simulink model "basic_model_2"  (R2024b)
settings: Solver=VariableStepAuto  StartTime=0.0  StopTime=0.2  RelTol=1e-3
libraries: spsPermanentMagnetSynchronousMachineLib x1, spsDCVoltageSourceLib x1, spsGroundLib x1, spsUniversalBridgeLib x1, sps_lib x1

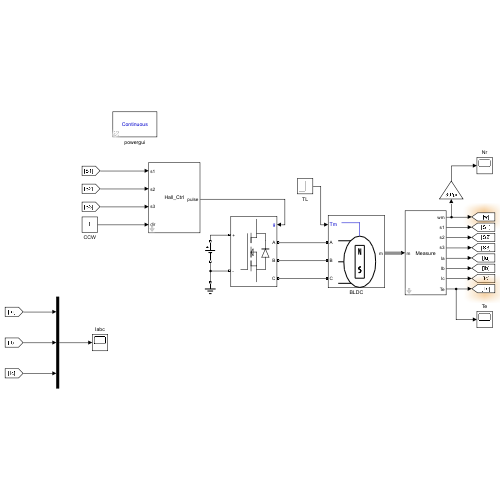
[thumbnail: Simulink's stored preview of the top-level diagram]
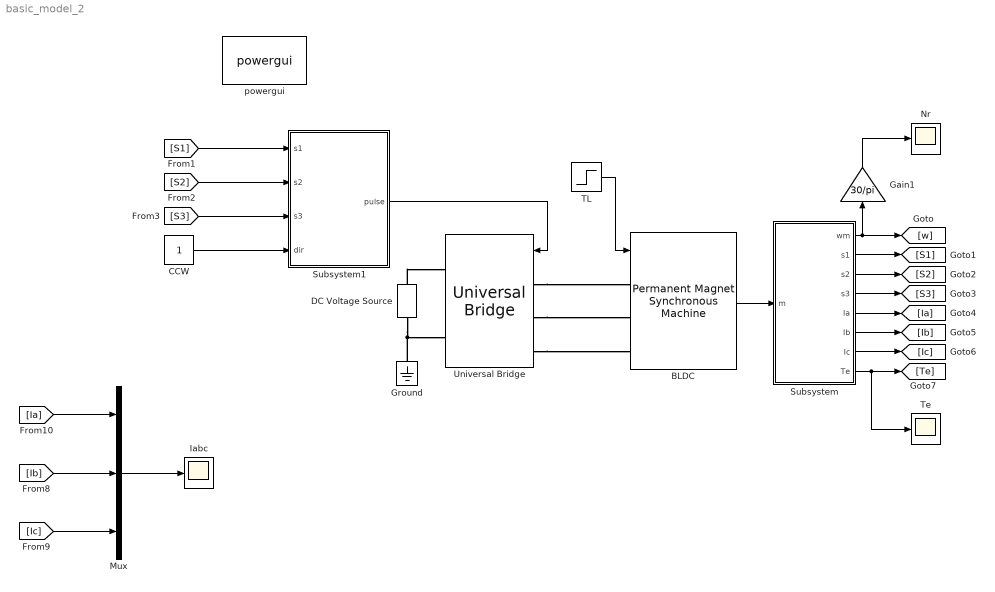
== system basic_model_2 ==
  BLDC : spsPermanentMagnetSynchronousMachineLib/Permanent Magnet Synchronous Machine  NbPhases=3  FluxDistribution=Trapezoidal  RotorType=Round  MechanicalLoad=Torque Tm  PresetModel=No  ShowDetailedParameters=on  MeasurementBus=off  Resistance=0.106/2  Inductance=0.000428/2  dqInductances=[8.5e-3,8.5e-3]  La=0.000395  MachineConstant=Torque Constant (N.m / A_peak)  Flux=0.041  VoltageCst=17.174  TorqueCst=0.164  Flat=120  Mechanical=[4943e-7 0.001 2 0]  PolePairs=4  InitialConditions=[0,0, 0,0]  InitialConditions5ph=[0 0 0 0 0 0]  RefAngle=Aligned with phase A axis (original Park)  IterativeDiscreteModel=Trapezoidal non iterative  TsBlock=-1  TsPowergui=0
  CCW : Constant
  DC Voltage Source : spsDCVoltageSourceLib/DC Voltage Source  Amplitude=50  Measurements=None
  Gain1 : Gain  Gain=30/pi
  Ground : spsGroundLib/Ground  LConnTagsString=a
  Iabc : Scope
  Mux : Mux  Inputs=3
  Nr : Scope
  Subsystem : Subsystem
  Subsystem1 : Subsystem
  TL : Step  Time=0.1  After=2  SampleTime=0
  Te : Scope
  Universal Bridge : spsUniversalBridgeLib/Universal Bridge  Arms=3  SnubberResistance=1e5  SnubberCapacitance=inf  Device=MOSFET / Diodes  Ron=1e-3  Lon=0  ForwardVoltages="[  0  0  ]"  ForwardVoltage=0  GTOparameters=[ 10e-6 , 20e-6 ]  IGBTparameters=[ 1e-6 , 2e-6 ]  Measurements=None  Measurements_2=None  converterType=Rectifier
  powergui : sps_lib/powergui  Priority=1  SimulationMode=Continuous  SampleTime=50e-6  frequency=60  Iterations=50  frequencyindice=0  Pbase=100e6  ErrMax=1e-4  UnitsV=kV  UnitsW=MW  buscounter=0  FunctionMessages=off  echomessages=off  EnableUseOfTLC=off  CurrentSourceSwitches=off  DisableSnubberDevices=off  DisableRonSwitches=off  DisableVfSwitches=off  DisplayEquations=off  AutomaticDiscreteSolvers=off  SolverType=Tustin/Backward Euler (TBE)  Interpol=off  ExternalGateDelay=off  methode=off  Ts=100  x0status=blocks  SPID=on  SwTol=0  HookPort=off  NonlinearTolerance=1e-4  nMaxIteration=100  ContinueOnMaxIteration=off  RestoreLinks=warning  ResistiveCurrentMeasurement=off  Frange=[0:2:500]  Ylog=off  Xlog=on  ShowGrid=off  save=off  variable=ZData  structure=0  ZoomFFT=off  StartTime=0.0  cycles=1  DisplayStyle=1  fundamental=60  FreqAxis=off  MaxFrequency=1000  frequencyindicesteady=1  RmsSteady=1  display=off
  wires:
  Mux/1 -> Iabc/1
  [Ic] -> Mux/3
  [Ia] -> Mux/1
  [Ib] -> Mux/2
  TL/1 -> BLDC/1
  BLDC/1 -> Subsystem/1(m)
  Subsystem/6(Ib) -> [Ib]
  Subsystem/2(s1) -> [S1]
  Subsystem/5(Ia) -> [Ia]
  Subsystem/7(Ic) -> [Ic]
  Subsystem/8(Te) -> Te/1, [Te]
  Subsystem/1(wm) -> Gain1/1, [w]
  Subsystem/3(s2) -> [S2]
  Gain1/1 -> Nr/1
  Subsystem/4(s3) -> [S3]
  [S1] -> Subsystem1/1(s1)
  [S2] -> Subsystem1/2(s2)
  [S3] -> Subsystem1/3(s3)
  CCW/1 -> Subsystem1/4(dir)
  Subsystem1/1(pulse) -> Universal Bridge/1
  connections:
  Universal Bridge/LConn3 -- BLDC/LConn3
  Universal Bridge/LConn2 -- BLDC/LConn2
  Universal Bridge/LConn1 -- BLDC/LConn1
  DC Voltage Source/RConn1 -- Universal Bridge/RConn1
  DC Voltage Source/LConn1 -- Ground/LConn1 -- Universal Bridge/RConn2

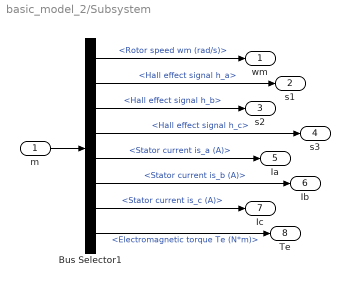
== system basic_model_2/Subsystem ==
  m : Inport
  Bus Selector1 : BusSelector  OutputSignals=Rotor speed wm (rad/s),Hall effect signal h_a,Hall effect signal h_b,Hall effect signal h_c,Stator current is_a (A),Stator current is_b (A),Stator current is_c (A),Electromagnetic torque Te (N*m)
  wm : Outport
  s1 : Outport  Port=2
  s2 : Outport  Port=3
  s3 : Outport  Port=4
  Ia : Outport  Port=5
  Ib : Outport  Port=6
  Ic : Outport  Port=7
  Te : Outport  Port=8
  wires:
  m/1 -> Bus Selector1/1
  Bus Selector1/5 -> Ia/1  "<Stator current is_a (A)>"
  Bus Selector1/8 -> Te/1  "<Electromagnetic torque Te (N*m)>"
  Bus Selector1/6 -> Ib/1  "<Stator current is_b (A)>"
  Bus Selector1/7 -> Ic/1  "<Stator current is_c (A)>"
  Bus Selector1/1 -> wm/1  "<Rotor speed wm (rad/s)>"
  Bus Selector1/2 -> s1/1  "<Hall effect signal h_a>"
  Bus Selector1/3 -> s2/1  "<Hall effect signal h_b>"
  Bus Selector1/4 -> s3/1  "<Hall effect signal h_c>"

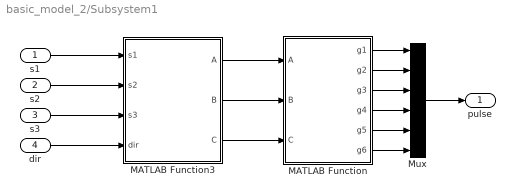
== system basic_model_2/Subsystem1 ==
  s1 : Inport
  s2 : Inport  Port=2
  s3 : Inport  Port=3
  dir : Inport  Port=4
  MATLAB Function : MATLAB Function  TreatAsAtomicUnit=on
  MATLAB Function3 : MATLAB Function  TreatAsAtomicUnit=on
  Mux : Mux  Inputs=6
  pulse : Outport
  wires:
  s2/1 -> MATLAB Function3/2(s2)
  MATLAB Function3/3(C) -> MATLAB Function/3(C)
  MATLAB Function3/2(B) -> MATLAB Function/2(B)
  MATLAB Function3/1(A) -> MATLAB Function/1(A)
  dir/1 -> MATLAB Function3/4(dir)
  s1/1 -> MATLAB Function3/1(s1)
  s3/1 -> MATLAB Function3/3(s3)
  MATLAB Function/1(g1) -> Mux/1
  MATLAB Function/2(g2) -> Mux/2
  MATLAB Function/3(g3) -> Mux/3
  MATLAB Function/4(g4) -> Mux/4
  MATLAB Function/5(g5) -> Mux/5
  MATLAB Function/6(g6) -> Mux/6
  Mux/1 -> pulse/1

== matlab function basic_model_2/Subsystem1/MATLAB Function3 ==
function [A,B,C] = Hall_Table(s1,s2,s3,dir)
    states = s1*4 + s2*2 + s3*1;
    if states == 0 || states == 7
        A = 0;
        B = 0;
        C = 0; % error Hall signals, stop motor
        return;
    end
    %map table
    map_tab = [6, 4, 5, 2, 1, 3];
    six_commut_tab = [1,-1,0; 1,0,-1;0,1,-1;-1,1,0;-1,0,1;0,-1,1];
    if dir > 0 %CCW, forward rotation
        index = map_tab(states);
    else %CW, reversal rotation
        index = mod(map_tab(states) - 1 + 3,6) + 1;
    end
    A = six_commut_tab(index,1);
    B = six_commut_tab(index,2);
    C = six_commut_tab(index,3);
end

== matlab function basic_model_2/Subsystem1/MATLAB Function ==
function [g1,g2,g3,g4,g5,g6] = Hall_pulse(A,B,C)
states = A*4 + B*2 + C*1;
pulse = [0,0,0,0,0,0];
if states == 0 || states == 7
    g1 = pulse(1);
    g2 = pulse(2);
    g3 = pulse(3);
    g4 = pulse(4);
    g5 = pulse(5);
    g6 = pulse(6);
    return;
end

if A == 0
    if B > 0
        pulse = [0,0,1,0,0,1];
    else
        pulse = [0,0,0,1,1,0];
    end
elseif B == 0
    if A > 0
        pulse = [1,0,0,0,0,1];
    else
        pulse = [0,1,0,0,1,0];
    end
elseif C == 0
    if A > 0
        pulse = [1,0,0,1,0,0];
    else
        pulse = [0,1,1,0,0,0];
    end
end
g1 = pulse(1);
g2 = pulse(2);
g3 = pulse(3);
g4 = pulse(4);
g5 = pulse(5);
g6 = pulse(6);
end
